simulink model "testing"  (R2017a)
settings: Solver=FixedStepAuto  StartTime=0.0  StopTime=inf  RelTol=1e-3  EnableMultiTasking=on
libraries: simulink x6, hdlsllib x5
settings Model: Creator=hyang344  LastModifiedBy=hyang344
settings SolverCC: AutoInsertRateTranBlk=on
settings OptimizationCC: BlockReduction=off  ConditionallyExecuteInputs=off  DefaultParameterBehavior=Inlined
settings DebuggingCC: AlgebraicLoopMsg=error  SingleTaskRateTransMsg=error
settings HardwareCC: ProdBitPerPointer=32  ProdBitPerSizeT=32  ProdBitPerPtrDiffT=32  ProdLargestAtomicFloat=None  ProdIntDivRoundTo=Undefined  ProdEndianess=Unspecified  ProdWordSize=32  ProdHWDeviceType=ASIC/FPGA->ASIC/FPGA  ProdEqTarget=off

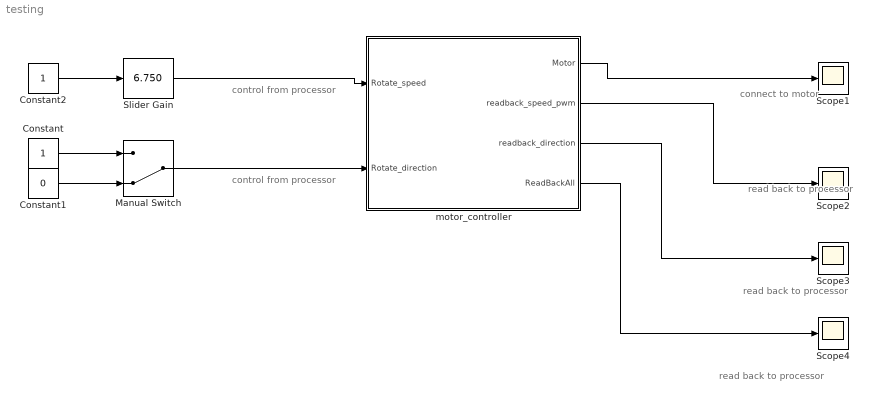
== system testing ==
  note: control from
      | processor
  note: read back to
      | processor
  note: control from
      | processor
  note: connect to
      | motor
  note: read back to
      | processor
  note: read back to
      | processor
  Constant : Constant  OutDataTypeStr=boolean
  Constant1 : Constant  Value=0  OutDataTypeStr=boolean
  Constant2 : Constant  OutDataTypeStr=fixdt(0, 4, 0)  SampleTime=0.1
  Manual Switch : ManualSwitch  CurrentSetting=0
  Scope{1..4} (4 alike) : Scope
  Slider Gain : simulink/Math Operations/Slider Gain  gain=6.750  low=0  high=15
  motor_controller : Subsystem  TreatAsAtomicUnit=on
  wires:
  Constant1/1 -> Manual Switch/2
  Slider Gain/1 -> motor_controller/1(Rotate_speed)
  Constant2/1 -> Slider Gain/1
  motor_controller/1(Motor) -> Scope1/1
  Constant/1 -> Manual Switch/1
  Manual Switch/1 -> motor_controller/2(Rotate_direction)
  motor_controller/2(readback_speed_pwm) -> Scope2/1
  motor_controller/3("readback_direction ") -> Scope3/1
  motor_controller/4(ReadBackAll) -> Scope4/1

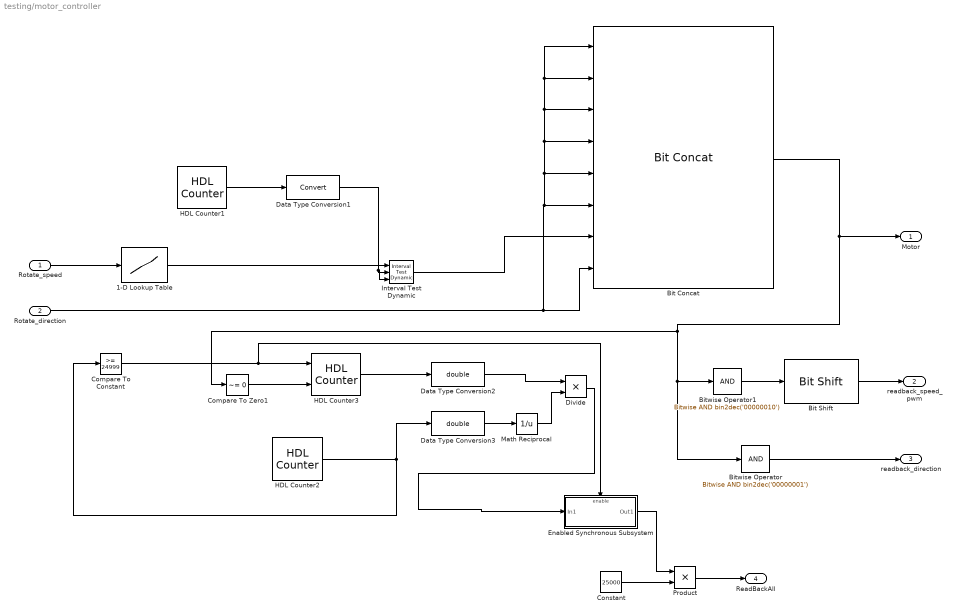
== system testing/motor_controller ==
  Rotate_speed : Inport  OutDataTypeStr=fixdt(0, 4, 0)
  Rotate_direction : Inport  Port=2  OutDataTypeStr=boolean
  1-D Lookup Table : Lookup_n-D  NumberOfTableDimensions=1  BreakpointsForDimension1=[0:15]  IndexSearchMethod=Evenly spaced points  Table=25000 * [0.25:0.05:1]  TableDataTypeStr=fixdt(0, 24, 0)  InterpMethod=Flat  DiagnosticForOutOfRangeInput=Error  OutDataTypeStr=fixdt(0, 24, 0)  RndMeth=Simplest  InputSameDT=on
  Bit Concat : hdlsllib/HDL Operations/Bit Concat  numInputs=8
      settings: SourceProductName=HDL Coder  SourceProductBaseCode=HD
  Bit Shift : hdlsllib/HDL Operations/Bit Shift  mode=Shift Right Logical  N=1
      settings: SourceProductName=HDL Coder  SourceProductBaseCode=HD
  Bitwise Operator : simulink/Logic and Bit Operations/Bitwise Operator  logicop=AND  UseBitMask=on  BitMask=bin2dec('00000001')  BitMaskRealWorld=Stored Integer
  Bitwise Operator1 : simulink/Logic and Bit Operations/Bitwise Operator  logicop=AND  UseBitMask=on  BitMask=bin2dec('00000010')  BitMaskRealWorld=Stored Integer
  Compare To Constant : simulink/Logic and Bit Operations/Compare To Constant  relop=>=  const=24999  OutDataTypeStr=boolean
  Compare To Zero1 : simulink/Logic and Bit Operations/Compare To Zero  relop=~=  OutDataTypeStr=boolean
  Constant : Constant  Value=25000  SampleTime=0.1
  Data Type Conversion1 : DataTypeConversion
  Data Type Conversion2 : DataTypeConversion  OutDataTypeStr=double
  Data Type Conversion3 : DataTypeConversion  OutDataTypeStr=double
  Divide : Product
  Enabled Synchronous Subsystem : Subsystem  TreatAsAtomicUnit=on
  HDL Counter1 : hdlsllib/HDL Operations/HDL Counter  CountType=Count limited  CountInit=0  CountStep=1  CountMax=25000  CountFromType=Initial value  CountFrom=0  CountResetPort=off  CountLoadPort=off  CountEnbPort=off  CountDirPort=off  CountDataType=Unsigned  CountWordLen=16  CountFracLen=0  CountSampTime=0.1
      settings: SourceProductName=HDL Coder  SourceProductBaseCode=HD
  HDL Counter2 : hdlsllib/HDL Operations/HDL Counter  CountType=Count limited  CountInit=0  CountStep=1  CountMax=25000  CountFromType=Initial value  CountFrom=0  CountResetPort=off  CountLoadPort=off  CountEnbPort=off  CountDirPort=off  CountDataType=Unsigned  CountWordLen=16  CountFracLen=0  CountSampTime=0.1
      settings: SourceProductName=HDL Coder  SourceProductBaseCode=HD
  HDL Counter3 : hdlsllib/HDL Operations/HDL Counter  CountType=Count limited  CountInit=0  CountStep=1  CountMax=25000  CountFromType=Initial value  CountFrom=0  CountResetPort=on  CountLoadPort=off  CountEnbPort=on  CountDirPort=off  CountDataType=Unsigned  CountWordLen=16  CountFracLen=0  CountSampTime=0.1
      settings: SourceProductName=HDL Coder  SourceProductBaseCode=HD
  Interval Test Dynamic : simulink/Logic and Bit Operations/Interval Test Dynamic  IntervalClosedRight=on  IntervalClosedLeft=on  OutDataTypeStr=boolean
      settings: SourceProductName=Simulink  SourceProductBaseCode=SL
  Math Reciprocal : Math  Operator=reciprocal  SaturateOnIntegerOverflow=on
  Product : Product  OutDataTypeStr=uint16
  Motor : Outport
  readback_speed_pwm : Outport  Port=2
  "readback_direction " : Outport  Port=3
  ReadBackAll : Outport  Port=4
  wires:
  Rotate_speed/1 -> 1-D Lookup Table/1
  1-D Lookup Table/1 -> Interval Test Dynamic/1
  Rotate_direction/1 -> Bit Concat/1, Bit Concat/2, Bit Concat/3, Bit Concat/4, Bit Concat/5, Bit Concat/6, Bit Concat/8
  HDL Counter1/1 -> Data Type Conversion1/1
  Data Type Conversion1/1 -> Interval Test Dynamic/3, Interval Test Dynamic/2
  Interval Test Dynamic/1 -> Bit Concat/7
  Bit Shift/1 -> readback_speed_pwm/1
  Bitwise Operator/1 -> "readback_direction "/1
  Bitwise Operator1/1 -> Bit Shift/1
  HDL Counter2/1 -> Data Type Conversion3/1, Compare To Constant/1
  Compare To Zero1/1 -> HDL Counter3/2
  Bit Concat/1 -> Compare To Zero1/1, Bitwise Operator1/1, Bitwise Operator/1, Motor/1
  Math Reciprocal/1 -> Divide/2
  HDL Counter3/1 -> Data Type Conversion2/1
  Data Type Conversion3/1 -> Math Reciprocal/1
  Data Type Conversion2/1 -> Divide/1
  Compare To Constant/1 -> Enabled Synchronous Subsystem/Enable, HDL Counter3/1
  Divide/1 -> Enabled Synchronous Subsystem/1(In1)
  Constant/1 -> Product/2
  Enabled Synchronous Subsystem/1(Out1) -> Product/1
  Product/1 -> ReadBackAll/1

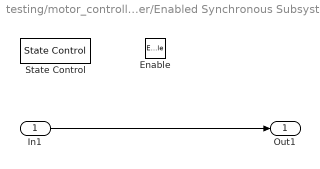
== system testing/motor_controller/Enabled Synchronous Subsystem ==
  In1 : Inport
  Enable : EnablePort
  State Control : StateControl  StateControl=Synchronous
  Out1 : Outport
  wires:
  In1/1 -> Out1/1
